simulink model "MODEL_FULL_SYSTEM"  (Simulink 7.8)
settings: Solver=ode1  StartTime=0.0  StopTime=inf  FixedStep=Ts  MaxStep=1e-3  RelTol=1e-3
PostLoadFcn:
  | Ts=80e-6; relays_settings_init;
InitFcn:
  | Ts=80e-6; relays_settings_init;
values from neighbouring files (symbols this model uses):
  relay_sets = xlsread('relay_settings_10272015.xlsx')    [relays_settings_init.m]
undefined symbols (not defined in the file or in its folder): dfilt, DiscIntNeverNeededParam, fdesignblkfcn, gcbh, Left, opmodbus_cb, ph, Right, type, V, X
libraries: simulink x72, modbus_lib x40, cables_lib x36, rtio_opalrt_common x21, rtlab x20, transformer_lib x13, dynamic_load_lib x12, powerlib x6, simulink_extras x6, ssn_lib x5, discretizing x4, rteventslib x4
(part 3 of 7)

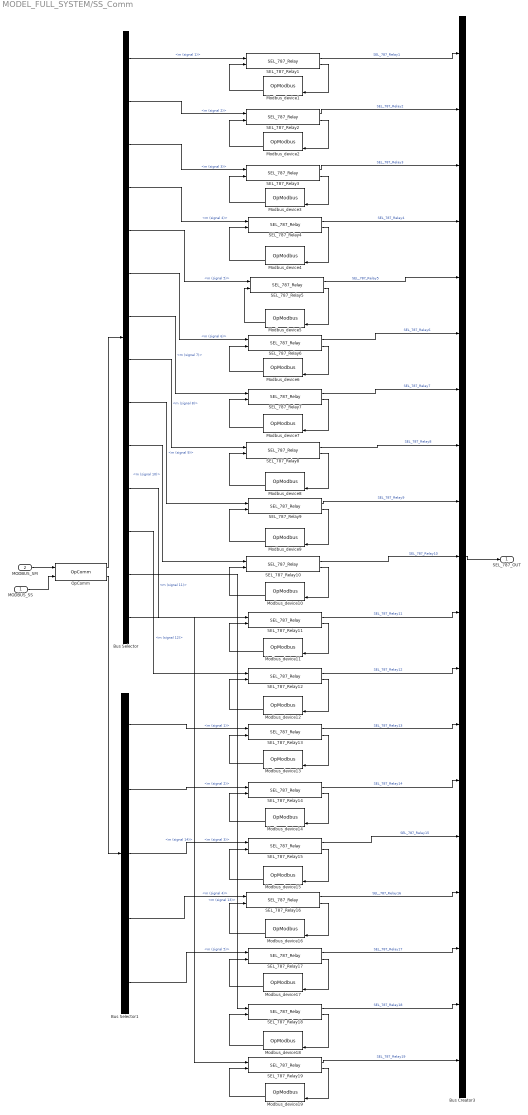
== system MODEL_FULL_SYSTEM/SS_Comm ==
  MODBUS_SS : Inport
  MODBUS_SM : Inport  Port=2
  Bus Creator3 : BusCreator  Inputs=19
  Bus Selector : BusSelector  OutputSignals=m (signal 1),m (signal 2),m (signal 3),m (signal 4),m (signal 5),m (signal 6),m (signal 7),m (signal 8),m (signal 9),m (signal 10),m (signal 11),m (signal 12),m (signal 13),m (signal 14)
  Bus Selector1 : BusSelector  OutputSignals=m (signal 1),m (signal 2),m (signal 3),m (signal 4),m (signal 5)
  Modbus_device1 : S-Function  InitFcn=opmodbus_cb();  FunctionName=OpModbus  Parameters=sample_time, conf_name  EnableBusSupport=off  mask(OpModbus){conf_name=relay_slave_cfg1.opal, conf_name_mask=relay_slave_cfg1.xls, sample_time=Ts}
      mask prompts: conf_name "Configuration file (OPAL)"; conf_name_mask "Configuration file"; sample_time "Sample time"
      mask help:
      | This block is used to simulate a Modbus-TCP Slave device. It allows exchanging data with any Modbus-TCP Master through Modbus Ethernet messaging. Using a standard network interface board, this block can be easily added to any simulation model.
      | All the configuration parameters are specified with a .csv or .xls 97-2003 file. This way, many parameters can be adjusted without re-compiling the model.
      | In real-time simulation mode, the complete modbus communication stack is handled by a dedicated thread running in parallel with the model. The communication stack does not add any significant or non-deterministic delay to the simulation.
      mask Help: eval('rtlab_io_help(''Generic/Modbus/OpModbus.htm'');');
      mask CallbackString: |opmodbus_cfg_cb('conf_name');|
      mask Display: disp(sprintf('Modbus'));
  Modbus_device10 : S-Function  InitFcn=opmodbus_cb();  FunctionName=OpModbus  Parameters=sample_time, conf_name  EnableBusSupport=off  mask(OpModbus){conf_name=relay_slave_cfg10.opal, conf_name_mask=relay_slave_cfg10.xls, sample_time=Ts}
      mask prompts: conf_name "Configuration file (OPAL)"; conf_name_mask "Configuration file"; sample_time "Sample time"
      mask help:
      | This block is used to simulate a Modbus-TCP Slave device. It allows exchanging data with any Modbus-TCP Master through Modbus Ethernet messaging. Using a standard network interface board, this block can be easily added to any simulation model.
      | All the configuration parameters are specified with a .csv or .xls 97-2003 file. This way, many parameters can be adjusted without re-compiling the model.
      | In real-time simulation mode, the complete modbus communication stack is handled by a dedicated thread running in parallel with the model. The communication stack does not add any significant or non-deterministic delay to the simulation.
      mask Help: eval('rtlab_io_help(''Generic/Modbus/OpModbus.htm'');');
      mask CallbackString: |opmodbus_cfg_cb('conf_name');|
      mask Display: disp(sprintf('Modbus'));
  Modbus_device11 : S-Function  InitFcn=opmodbus_cb();  FunctionName=OpModbus  Parameters=sample_time, conf_name  EnableBusSupport=off  mask(OpModbus){conf_name=relay_slave_cfg11.opal, conf_name_mask=relay_slave_cfg11.xls, sample_time=Ts}
      mask prompts: conf_name "Configuration file (OPAL)"; conf_name_mask "Configuration file"; sample_time "Sample time"
      mask help:
      | This block is used to simulate a Modbus-TCP Slave device. It allows exchanging data with any Modbus-TCP Master through Modbus Ethernet messaging. Using a standard network interface board, this block can be easily added to any simulation model.
      | All the configuration parameters are specified with a .csv or .xls 97-2003 file. This way, many parameters can be adjusted without re-compiling the model.
      | In real-time simulation mode, the complete modbus communication stack is handled by a dedicated thread running in parallel with the model. The communication stack does not add any significant or non-deterministic delay to the simulation.
      mask Help: eval('rtlab_io_help(''Generic/Modbus/OpModbus.htm'');');
      mask CallbackString: |opmodbus_cfg_cb('conf_name');|
      mask Display: disp(sprintf('Modbus'));
  Modbus_device12 : S-Function  InitFcn=opmodbus_cb();  FunctionName=OpModbus  Parameters=sample_time, conf_name  EnableBusSupport=off  mask(OpModbus){conf_name=relay_slave_cfg12.opal, conf_name_mask=relay_slave_cfg12.xls, sample_time=Ts}
      mask prompts: conf_name "Configuration file (OPAL)"; conf_name_mask "Configuration file"; sample_time "Sample time"
      mask help:
      | This block is used to simulate a Modbus-TCP Slave device. It allows exchanging data with any Modbus-TCP Master through Modbus Ethernet messaging. Using a standard network interface board, this block can be easily added to any simulation model.
      | All the configuration parameters are specified with a .csv or .xls 97-2003 file. This way, many parameters can be adjusted without re-compiling the model.
      | In real-time simulation mode, the complete modbus communication stack is handled by a dedicated thread running in parallel with the model. The communication stack does not add any significant or non-deterministic delay to the simulation.
      mask Help: eval('rtlab_io_help(''Generic/Modbus/OpModbus.htm'');');
      mask CallbackString: |opmodbus_cfg_cb('conf_name');|
      mask Display: disp(sprintf('Modbus'));
  Modbus_device13 : S-Function  InitFcn=opmodbus_cb();  FunctionName=OpModbus  Parameters=sample_time, conf_name  EnableBusSupport=off  mask(OpModbus){conf_name=relay_slave_cfg13.opal, conf_name_mask=relay_slave_cfg13.xls, sample_time=Ts}
      mask prompts: conf_name "Configuration file (OPAL)"; conf_name_mask "Configuration file"; sample_time "Sample time"
      mask help:
      | This block is used to simulate a Modbus-TCP Slave device. It allows exchanging data with any Modbus-TCP Master through Modbus Ethernet messaging. Using a standard network interface board, this block can be easily added to any simulation model.
      | All the configuration parameters are specified with a .csv or .xls 97-2003 file. This way, many parameters can be adjusted without re-compiling the model.
      | In real-time simulation mode, the complete modbus communication stack is handled by a dedicated thread running in parallel with the model. The communication stack does not add any significant or non-deterministic delay to the simulation.
      mask Help: eval('rtlab_io_help(''Generic/Modbus/OpModbus.htm'');');
      mask CallbackString: |opmodbus_cfg_cb('conf_name');|
      mask Display: disp(sprintf('Modbus'));
  Modbus_device14 : S-Function  InitFcn=opmodbus_cb();  FunctionName=OpModbus  Parameters=sample_time, conf_name  EnableBusSupport=off  mask(OpModbus){conf_name=relay_slave_cfg14.opal, conf_name_mask=relay_slave_cfg14.xls, sample_time=Ts}
      mask prompts: conf_name "Configuration file (OPAL)"; conf_name_mask "Configuration file"; sample_time "Sample time"
      mask help:
      | This block is used to simulate a Modbus-TCP Slave device. It allows exchanging data with any Modbus-TCP Master through Modbus Ethernet messaging. Using a standard network interface board, this block can be easily added to any simulation model.
      | All the configuration parameters are specified with a .csv or .xls 97-2003 file. This way, many parameters can be adjusted without re-compiling the model.
      | In real-time simulation mode, the complete modbus communication stack is handled by a dedicated thread running in parallel with the model. The communication stack does not add any significant or non-deterministic delay to the simulation.
      mask Help: eval('rtlab_io_help(''Generic/Modbus/OpModbus.htm'');');
      mask CallbackString: |opmodbus_cfg_cb('conf_name');|
      mask Display: disp(sprintf('Modbus'));
  Modbus_device15 : S-Function  InitFcn=opmodbus_cb();  FunctionName=OpModbus  Parameters=sample_time, conf_name  EnableBusSupport=off  mask(OpModbus){conf_name=relay_slave_cfg15.opal, conf_name_mask=relay_slave_cfg15.xls, sample_time=Ts}
      mask prompts: conf_name "Configuration file (OPAL)"; conf_name_mask "Configuration file"; sample_time "Sample time"
      mask help:
      | This block is used to simulate a Modbus-TCP Slave device. It allows exchanging data with any Modbus-TCP Master through Modbus Ethernet messaging. Using a standard network interface board, this block can be easily added to any simulation model.
      | All the configuration parameters are specified with a .csv or .xls 97-2003 file. This way, many parameters can be adjusted without re-compiling the model.
      | In real-time simulation mode, the complete modbus communication stack is handled by a dedicated thread running in parallel with the model. The communication stack does not add any significant or non-deterministic delay to the simulation.
      mask Help: eval('rtlab_io_help(''Generic/Modbus/OpModbus.htm'');');
      mask CallbackString: |opmodbus_cfg_cb('conf_name');|
      mask Display: disp(sprintf('Modbus'));
  Modbus_device16 : S-Function  InitFcn=opmodbus_cb();  FunctionName=OpModbus  Parameters=sample_time, conf_name  EnableBusSupport=off  mask(OpModbus){conf_name=relay_slave_cfg16.opal, conf_name_mask=relay_slave_cfg16.xls, sample_time=Ts}
      mask prompts: conf_name "Configuration file (OPAL)"; conf_name_mask "Configuration file"; sample_time "Sample time"
      mask help:
      | This block is used to simulate a Modbus-TCP Slave device. It allows exchanging data with any Modbus-TCP Master through Modbus Ethernet messaging. Using a standard network interface board, this block can be easily added to any simulation model.
      | All the configuration parameters are specified with a .csv or .xls 97-2003 file. This way, many parameters can be adjusted without re-compiling the model.
      | In real-time simulation mode, the complete modbus communication stack is handled by a dedicated thread running in parallel with the model. The communication stack does not add any significant or non-deterministic delay to the simulation.
      mask Help: eval('rtlab_io_help(''Generic/Modbus/OpModbus.htm'');');
      mask CallbackString: |opmodbus_cfg_cb('conf_name');|
      mask Display: disp(sprintf('Modbus'));
  Modbus_device17 : S-Function  InitFcn=opmodbus_cb();  FunctionName=OpModbus  Parameters=sample_time, conf_name  EnableBusSupport=off  mask(OpModbus){conf_name=relay_slave_cfg17.opal, conf_name_mask=relay_slave_cfg17.xls, sample_time=Ts}
      mask prompts: conf_name "Configuration file (OPAL)"; conf_name_mask "Configuration file"; sample_time "Sample time"
      mask help:
      | This block is used to simulate a Modbus-TCP Slave device. It allows exchanging data with any Modbus-TCP Master through Modbus Ethernet messaging. Using a standard network interface board, this block can be easily added to any simulation model.
      | All the configuration parameters are specified with a .csv or .xls 97-2003 file. This way, many parameters can be adjusted without re-compiling the model.
      | In real-time simulation mode, the complete modbus communication stack is handled by a dedicated thread running in parallel with the model. The communication stack does not add any significant or non-deterministic delay to the simulation.
      mask Help: eval('rtlab_io_help(''Generic/Modbus/OpModbus.htm'');');
      mask CallbackString: |opmodbus_cfg_cb('conf_name');|
      mask Display: disp(sprintf('Modbus'));
  Modbus_device18 : S-Function  InitFcn=opmodbus_cb();  FunctionName=OpModbus  Parameters=sample_time, conf_name  EnableBusSupport=off  mask(OpModbus){conf_name=relay_slave_cfg18.opal, conf_name_mask=relay_slave_cfg18.xls, sample_time=Ts}
      mask prompts: conf_name "Configuration file (OPAL)"; conf_name_mask "Configuration file"; sample_time "Sample time"
      mask help:
      | This block is used to simulate a Modbus-TCP Slave device. It allows exchanging data with any Modbus-TCP Master through Modbus Ethernet messaging. Using a standard network interface board, this block can be easily added to any simulation model.
      | All the configuration parameters are specified with a .csv or .xls 97-2003 file. This way, many parameters can be adjusted without re-compiling the model.
      | In real-time simulation mode, the complete modbus communication stack is handled by a dedicated thread running in parallel with the model. The communication stack does not add any significant or non-deterministic delay to the simulation.
      mask Help: eval('rtlab_io_help(''Generic/Modbus/OpModbus.htm'');');
      mask CallbackString: |opmodbus_cfg_cb('conf_name');|
      mask Display: disp(sprintf('Modbus'));
  Modbus_device19 : S-Function  InitFcn=opmodbus_cb();  FunctionName=OpModbus  Parameters=sample_time, conf_name  EnableBusSupport=off  mask(OpModbus){conf_name=relay_slave_cfg19.opal, conf_name_mask=relay_slave_cfg19.xls, sample_time=Ts}
      mask prompts: conf_name "Configuration file (OPAL)"; conf_name_mask "Configuration file"; sample_time "Sample time"
      mask help:
      | This block is used to simulate a Modbus-TCP Slave device. It allows exchanging data with any Modbus-TCP Master through Modbus Ethernet messaging. Using a standard network interface board, this block can be easily added to any simulation model.
      | All the configuration parameters are specified with a .csv or .xls 97-2003 file. This way, many parameters can be adjusted without re-compiling the model.
      | In real-time simulation mode, the complete modbus communication stack is handled by a dedicated thread running in parallel with the model. The communication stack does not add any significant or non-deterministic delay to the simulation.
      mask Help: eval('rtlab_io_help(''Generic/Modbus/OpModbus.htm'');');
      mask CallbackString: |opmodbus_cfg_cb('conf_name');|
      mask Display: disp(sprintf('Modbus'));
  Modbus_device2 : S-Function  InitFcn=opmodbus_cb();  FunctionName=OpModbus  Parameters=sample_time, conf_name  EnableBusSupport=off  mask(OpModbus){conf_name=relay_slave_cfg2.opal, conf_name_mask=relay_slave_cfg2.xls, sample_time=Ts}
      mask prompts: conf_name "Configuration file (OPAL)"; conf_name_mask "Configuration file"; sample_time "Sample time"
      mask help:
      | This block is used to simulate a Modbus-TCP Slave device. It allows exchanging data with any Modbus-TCP Master through Modbus Ethernet messaging. Using a standard network interface board, this block can be easily added to any simulation model.
      | All the configuration parameters are specified with a .csv or .xls 97-2003 file. This way, many parameters can be adjusted without re-compiling the model.
      | In real-time simulation mode, the complete modbus communication stack is handled by a dedicated thread running in parallel with the model. The communication stack does not add any significant or non-deterministic delay to the simulation.
      mask Help: eval('rtlab_io_help(''Generic/Modbus/OpModbus.htm'');');
      mask CallbackString: |opmodbus_cfg_cb('conf_name');|
      mask Display: disp(sprintf('Modbus'));
  Modbus_device3 : S-Function  InitFcn=opmodbus_cb();  FunctionName=OpModbus  Parameters=sample_time, conf_name  EnableBusSupport=off  mask(OpModbus){conf_name=relay_slave_cfg3.opal, conf_name_mask=relay_slave_cfg3.xls, sample_time=Ts}
      mask prompts: conf_name "Configuration file (OPAL)"; conf_name_mask "Configuration file"; sample_time "Sample time"
      mask help:
      | This block is used to simulate a Modbus-TCP Slave device. It allows exchanging data with any Modbus-TCP Master through Modbus Ethernet messaging. Using a standard network interface board, this block can be easily added to any simulation model.
      | All the configuration parameters are specified with a .csv or .xls 97-2003 file. This way, many parameters can be adjusted without re-compiling the model.
      | In real-time simulation mode, the complete modbus communication stack is handled by a dedicated thread running in parallel with the model. The communication stack does not add any significant or non-deterministic delay to the simulation.
      mask Help: eval('rtlab_io_help(''Generic/Modbus/OpModbus.htm'');');
      mask CallbackString: |opmodbus_cfg_cb('conf_name');|
      mask Display: disp(sprintf('Modbus'));
  Modbus_device4 : S-Function  InitFcn=opmodbus_cb();  FunctionName=OpModbus  Parameters=sample_time, conf_name  EnableBusSupport=off  mask(OpModbus){conf_name=relay_slave_cfg4.opal, conf_name_mask=relay_slave_cfg4.xls, sample_time=Ts}
      mask prompts: conf_name "Configuration file (OPAL)"; conf_name_mask "Configuration file"; sample_time "Sample time"
      mask help:
      | This block is used to simulate a Modbus-TCP Slave device. It allows exchanging data with any Modbus-TCP Master through Modbus Ethernet messaging. Using a standard network interface board, this block can be easily added to any simulation model.
      | All the configuration parameters are specified with a .csv or .xls 97-2003 file. This way, many parameters can be adjusted without re-compiling the model.
      | In real-time simulation mode, the complete modbus communication stack is handled by a dedicated thread running in parallel with the model. The communication stack does not add any significant or non-deterministic delay to the simulation.
      mask Help: eval('rtlab_io_help(''Generic/Modbus/OpModbus.htm'');');
      mask CallbackString: |opmodbus_cfg_cb('conf_name');|
      mask Display: disp(sprintf('Modbus'));
  Modbus_device5 : S-Function  InitFcn=opmodbus_cb();  FunctionName=OpModbus  Parameters=sample_time, conf_name  EnableBusSupport=off  mask(OpModbus){conf_name=relay_slave_cfg5.opal, conf_name_mask=relay_slave_cfg5.xls, sample_time=Ts}
      mask prompts: conf_name "Configuration file (OPAL)"; conf_name_mask "Configuration file"; sample_time "Sample time"
      mask help:
      | This block is used to simulate a Modbus-TCP Slave device. It allows exchanging data with any Modbus-TCP Master through Modbus Ethernet messaging. Using a standard network interface board, this block can be easily added to any simulation model.
      | All the configuration parameters are specified with a .csv or .xls 97-2003 file. This way, many parameters can be adjusted without re-compiling the model.
      | In real-time simulation mode, the complete modbus communication stack is handled by a dedicated thread running in parallel with the model. The communication stack does not add any significant or non-deterministic delay to the simulation.
      mask Help: eval('rtlab_io_help(''Generic/Modbus/OpModbus.htm'');');
      mask CallbackString: |opmodbus_cfg_cb('conf_name');|
      mask Display: disp(sprintf('Modbus'));
  Modbus_device6 : S-Function  InitFcn=opmodbus_cb();  FunctionName=OpModbus  Parameters=sample_time, conf_name  EnableBusSupport=off  mask(OpModbus){conf_name=relay_slave_cfg6.opal, conf_name_mask=relay_slave_cfg6.xls, sample_time=Ts}
      mask prompts: conf_name "Configuration file (OPAL)"; conf_name_mask "Configuration file"; sample_time "Sample time"
      mask help:
      | This block is used to simulate a Modbus-TCP Slave device. It allows exchanging data with any Modbus-TCP Master through Modbus Ethernet messaging. Using a standard network interface board, this block can be easily added to any simulation model.
      | All the configuration parameters are specified with a .csv or .xls 97-2003 file. This way, many parameters can be adjusted without re-compiling the model.
      | In real-time simulation mode, the complete modbus communication stack is handled by a dedicated thread running in parallel with the model. The communication stack does not add any significant or non-deterministic delay to the simulation.
      mask Help: eval('rtlab_io_help(''Generic/Modbus/OpModbus.htm'');');
      mask CallbackString: |opmodbus_cfg_cb('conf_name');|
      mask Display: disp(sprintf('Modbus'));
  Modbus_device7 : S-Function  InitFcn=opmodbus_cb();  FunctionName=OpModbus  Parameters=sample_time, conf_name  EnableBusSupport=off  mask(OpModbus){conf_name=relay_slave_cfg7.opal, conf_name_mask=relay_slave_cfg7.xls, sample_time=Ts}
      mask prompts: conf_name "Configuration file (OPAL)"; conf_name_mask "Configuration file"; sample_time "Sample time"
      mask help:
      | This block is used to simulate a Modbus-TCP Slave device. It allows exchanging data with any Modbus-TCP Master through Modbus Ethernet messaging. Using a standard network interface board, this block can be easily added to any simulation model.
      | All the configuration parameters are specified with a .csv or .xls 97-2003 file. This way, many parameters can be adjusted without re-compiling the model.
      | In real-time simulation mode, the complete modbus communication stack is handled by a dedicated thread running in parallel with the model. The communication stack does not add any significant or non-deterministic delay to the simulation.
      mask Help: eval('rtlab_io_help(''Generic/Modbus/OpModbus.htm'');');
      mask CallbackString: |opmodbus_cfg_cb('conf_name');|
      mask Display: disp(sprintf('Modbus'));
  Modbus_device8 : S-Function  InitFcn=opmodbus_cb();  FunctionName=OpModbus  Parameters=sample_time, conf_name  EnableBusSupport=off  mask(OpModbus){conf_name=relay_slave_cfg8.opal, conf_name_mask=relay_slave_cfg8.xls, sample_time=Ts}
      mask prompts: conf_name "Configuration file (OPAL)"; conf_name_mask "Configuration file"; sample_time "Sample time"
      mask help:
      | This block is used to simulate a Modbus-TCP Slave device. It allows exchanging data with any Modbus-TCP Master through Modbus Ethernet messaging. Using a standard network interface board, this block can be easily added to any simulation model.
      | All the configuration parameters are specified with a .csv or .xls 97-2003 file. This way, many parameters can be adjusted without re-compiling the model.
      | In real-time simulation mode, the complete modbus communication stack is handled by a dedicated thread running in parallel with the model. The communication stack does not add any significant or non-deterministic delay to the simulation.
      mask Help: eval('rtlab_io_help(''Generic/Modbus/OpModbus.htm'');');
      mask CallbackString: |opmodbus_cfg_cb('conf_name');|
      mask Display: disp(sprintf('Modbus'));
  Modbus_device9 : S-Function  InitFcn=opmodbus_cb();  FunctionName=OpModbus  Parameters=sample_time, conf_name  EnableBusSupport=off  mask(OpModbus){conf_name=relay_slave_cfg9.opal, conf_name_mask=relay_slave_cfg9.xls, sample_time=Ts}
      mask prompts: conf_name "Configuration file (OPAL)"; conf_name_mask "Configuration file"; sample_time "Sample time"
      mask help:
      | This block is used to simulate a Modbus-TCP Slave device. It allows exchanging data with any Modbus-TCP Master through Modbus Ethernet messaging. Using a standard network interface board, this block can be easily added to any simulation model.
      | All the configuration parameters are specified with a .csv or .xls 97-2003 file. This way, many parameters can be adjusted without re-compiling the model.
      | In real-time simulation mode, the complete modbus communication stack is handled by a dedicated thread running in parallel with the model. The communication stack does not add any significant or non-deterministic delay to the simulation.
      mask Help: eval('rtlab_io_help(''Generic/Modbus/OpModbus.htm'');');
      mask CallbackString: |opmodbus_cfg_cb('conf_name');|
      mask Display: disp(sprintf('Modbus'));
  OpComm : rtlab/OpComm  nbport=2  groupe_acq=1  subsys_rate=0  st=0  Synchronization=on  Interpolation=on  Threshold=1.0  Missed_Data=off  Sim_Time=off  Samples=off  dynSigOut=off  from_console=0  warning_done=off  writeOpCommFile=off  Offset=off
  SEL_787_Relay1 : modbus_lib/SEL_787_Relay  bkrCtrl_enable=0  bkrCtrl_status=1  settings=[relay_sets(1, :)]  Ts=Ts
  SEL_787_Relay10 : modbus_lib/SEL_787_Relay  bkrCtrl_enable=0  bkrCtrl_status=1  settings=[relay_sets(10, :)]  Ts=Ts
  SEL_787_Relay11 : modbus_lib/SEL_787_Relay  bkrCtrl_enable=0  bkrCtrl_status=1  settings=[relay_sets(11, :)]  Ts=Ts
  SEL_787_Relay12 : modbus_lib/SEL_787_Relay  bkrCtrl_enable=0  bkrCtrl_status=1  settings=[relay_sets(12, :)]  Ts=Ts
  SEL_787_Relay13 : modbus_lib/SEL_787_Relay  bkrCtrl_enable=0  bkrCtrl_status=1  settings=[relay_sets(13, :)]  Ts=Ts
  SEL_787_Relay14 : modbus_lib/SEL_787_Relay  bkrCtrl_enable=0  bkrCtrl_status=1  settings=[relay_sets(14, :)]  Ts=Ts
  SEL_787_Relay15 : modbus_lib/SEL_787_Relay  bkrCtrl_enable=0  bkrCtrl_status=1  settings=[relay_sets(15, :)]  Ts=Ts
  SEL_787_Relay16 : modbus_lib/SEL_787_Relay  bkrCtrl_enable=0  bkrCtrl_status=1  settings=[relay_sets(16, :)]  Ts=Ts
  SEL_787_Relay17 : modbus_lib/SEL_787_Relay  bkrCtrl_enable=0  bkrCtrl_status=1  settings=[relay_sets(17, :)]  Ts=Ts
  SEL_787_Relay18 : modbus_lib/SEL_787_Relay  bkrCtrl_enable=0  bkrCtrl_status=1  settings=[relay_sets(18, :)]  Ts=Ts
  SEL_787_Relay19 : modbus_lib/SEL_787_Relay  bkrCtrl_enable=0  bkrCtrl_status=1  settings=[relay_sets(19, :)]  Ts=Ts
  SEL_787_Relay2 : modbus_lib/SEL_787_Relay  bkrCtrl_enable=0  bkrCtrl_status=1  settings=[relay_sets(2, :)]  Ts=Ts
  SEL_787_Relay3 : modbus_lib/SEL_787_Relay  bkrCtrl_enable=0  bkrCtrl_status=1  settings=[relay_sets(3, :)]  Ts=Ts
  SEL_787_Relay4 : modbus_lib/SEL_787_Relay  bkrCtrl_enable=0  bkrCtrl_status=1  settings=[relay_sets(4, :)]  Ts=Ts
  SEL_787_Relay5 : modbus_lib/SEL_787_Relay  bkrCtrl_enable=0  bkrCtrl_status=1  settings=[relay_sets(5, :)]  Ts=Ts
  SEL_787_Relay6 : modbus_lib/SEL_787_Relay  bkrCtrl_enable=0  bkrCtrl_status=1  settings=[relay_sets(6, :)]  Ts=Ts
  SEL_787_Relay7 : modbus_lib/SEL_787_Relay  bkrCtrl_enable=0  bkrCtrl_status=1  settings=[relay_sets(7, :)]  Ts=Ts
  SEL_787_Relay8 : modbus_lib/SEL_787_Relay  bkrCtrl_enable=0  bkrCtrl_status=1  settings=[relay_sets(8, :)]  Ts=Ts
  SEL_787_Relay9 : modbus_lib/SEL_787_Relay  bkrCtrl_enable=0  bkrCtrl_status=1  settings=[relay_sets(9, :)]  Ts=Ts
  SEL_787_OUT : Outport
  wires:
  MODBUS_SM/1 -> OpComm/1
  OpComm/1 -> Bus Selector/1
  SEL_787_Relay1/1 -> Bus Creator3/1  "SEL_787_Relay1"
  Bus Creator3/1 -> SEL_787_OUT/1
  SEL_787_Relay10/1 -> Bus Creator3/10  "SEL_787_Relay10"
  SEL_787_Relay2/1 -> Bus Creator3/2  "SEL_787_Relay2"
  SEL_787_Relay3/1 -> Bus Creator3/3  "SEL_787_Relay3"
  SEL_787_Relay4/1 -> Bus Creator3/4  "SEL_787_Relay4"
  SEL_787_Relay5/1 -> Bus Creator3/5  "SEL_787_Relay5"
  SEL_787_Relay6/1 -> Bus Creator3/6  "SEL_787_Relay6"
  SEL_787_Relay9/1 -> Bus Creator3/9  "SEL_787_Relay9"
  SEL_787_Relay17/1 -> Bus Creator3/17  "SEL_787_Relay17"
  SEL_787_Relay11/1 -> Bus Creator3/11  "SEL_787_Relay11"
  SEL_787_Relay12/1 -> Bus Creator3/12  "SEL_787_Relay12"
  SEL_787_Relay13/1 -> Bus Creator3/13  "SEL_787_Relay13"
  SEL_787_Relay14/1 -> Bus Creator3/14  "SEL_787_Relay14"
  SEL_787_Relay15/1 -> Bus Creator3/15  "SEL_787_Relay15"
  SEL_787_Relay16/1 -> Bus Creator3/16  "SEL_787_Relay16"
  SEL_787_Relay7/1 -> Bus Creator3/7  "SEL_787_Relay7"
  SEL_787_Relay8/1 -> Bus Creator3/8  "SEL_787_Relay8"
  SEL_787_Relay18/1 -> Bus Creator3/18  "SEL_787_Relay18"
  SEL_787_Relay19/1 -> Bus Creator3/19  "SEL_787_Relay19"
  MODBUS_SS/1 -> OpComm/2
  OpComm/2 -> Bus Selector1/1
  Modbus_device1/2 -> SEL_787_Relay1/2
  SEL_787_Relay1/2 -> Modbus_device1/4
  SEL_787_Relay2/2 -> Modbus_device2/4
  Modbus_device2/2 -> SEL_787_Relay2/2
  SEL_787_Relay3/2 -> Modbus_device3/4
  Modbus_device3/2 -> SEL_787_Relay3/2
  SEL_787_Relay4/2 -> Modbus_device4/4
  Modbus_device4/2 -> SEL_787_Relay4/2
  Modbus_device5/2 -> SEL_787_Relay5/2
  SEL_787_Relay5/2 -> Modbus_device5/4
  Modbus_device6/2 -> SEL_787_Relay6/2
  SEL_787_Relay6/2 -> Modbus_device6/4
  SEL_787_Relay7/2 -> Modbus_device7/4
  Modbus_device7/2 -> SEL_787_Relay7/2
  Modbus_device8/2 -> SEL_787_Relay8/2
  SEL_787_Relay8/2 -> Modbus_device8/4
  SEL_787_Relay9/2 -> Modbus_device9/4
  Modbus_device9/2 -> SEL_787_Relay9/2
  SEL_787_Relay10/2 -> Modbus_device10/4
  Modbus_device10/2 -> SEL_787_Relay10/2
  Modbus_device11/2 -> SEL_787_Relay11/2
  SEL_787_Relay11/2 -> Modbus_device11/4
  SEL_787_Relay12/2 -> Modbus_device12/4
  Modbus_device12/2 -> SEL_787_Relay12/2
  Modbus_device13/2 -> SEL_787_Relay13/2
  SEL_787_Relay13/2 -> Modbus_device13/4
  SEL_787_Relay14/2 -> Modbus_device14/4
  Modbus_device14/2 -> SEL_787_Relay14/2
  Modbus_device15/2 -> SEL_787_Relay15/2
  SEL_787_Relay15/2 -> Modbus_device15/4
  SEL_787_Relay16/2 -> Modbus_device16/4
  Modbus_device16/2 -> SEL_787_Relay16/2
  Modbus_device17/2 -> SEL_787_Relay17/2
  SEL_787_Relay17/2 -> Modbus_device17/4
  SEL_787_Relay18/2 -> Modbus_device18/4
  Modbus_device18/2 -> SEL_787_Relay18/2
  Modbus_device19/2 -> SEL_787_Relay19/2
  SEL_787_Relay19/2 -> Modbus_device19/4
  Bus Selector/1 -> SEL_787_Relay1/1  "<m (signal 1)>"
  Bus Selector/2 -> SEL_787_Relay2/1  "<m (signal 2)>"
  Bus Selector/3 -> SEL_787_Relay3/1  "<m (signal 3)>"
  Bus Selector/4 -> SEL_787_Relay4/1  "<m (signal 4)>"
  Bus Selector/5 -> SEL_787_Relay5/1  "<m (signal 5)>"
  Bus Selector/6 -> SEL_787_Relay6/1  "<m (signal 6)>"
  Bus Selector/7 -> SEL_787_Relay7/1  "<m (signal 7)>"
  Bus Selector/8 -> SEL_787_Relay8/1  "<m (signal 8)>"
  Bus Selector/9 -> SEL_787_Relay9/1  "<m (signal 9)>"
  Bus Selector/10 -> SEL_787_Relay10/1  "<m (signal 10)>"
  Bus Selector/11 -> SEL_787_Relay11/1  "<m (signal 11)>"
  Bus Selector/12 -> SEL_787_Relay12/1  "<m (signal 12)>"
  Bus Selector1/1 -> SEL_787_Relay13/1  "<m (signal 1)>"
  Bus Selector1/2 -> SEL_787_Relay14/1  "<m (signal 2)>"
  Bus Selector1/3 -> SEL_787_Relay15/1  "<m (signal 3)>"
  Bus Selector1/4 -> SEL_787_Relay16/1  "<m (signal 4)>"
  Bus Selector1/5 -> SEL_787_Relay17/1  "<m (signal 5)>"
  Bus Selector/13 -> SEL_787_Relay18/1  "<m (signal 13)>"
  Bus Selector/14 -> SEL_787_Relay19/1  "<m (signal 14)>"
